simulink model "rlKinovaBallBalance"  (R2024a)
settings: Solver=ode15s  StartTime=0.0  StopTime=inf  MaxStep=0.005  RelTol=1e-4  AbsTol=1e-4
values from neighbouring files (symbols this model uses):
  max_torque = [3.5;    0.1;   0.75;    0.5]    [kinova_params.m]
  R1_q0 = 0    [kinova_params.m]
  R2_q0 = deg2rad(20)    [kinova_params.m]
  R3_q0 = 0    [kinova_params.m]
  R4_q0 = deg2rad(135)    [kinova_params.m]
  R5_q0 = 0    [kinova_params.m]
  R6_q0 = deg2rad(-65)    [kinova_params.m]
  R7_q0 = deg2rad(-90)    [kinova_params.m]
  U0 = [11.9 0.1 -1.4 0.09]    [kinova_params.m]
undefined symbols (not defined in the file or in its folder): Control, fluent0, L1, L2, L3, LS1, LS3, plate, R1, R2, R3, Rover, rover_path, RS1, RS3, Ts, vessel, X, Y, Z
libraries: sm_lib x253, nesl_utility x111, fl_lib x85, nesl_utility_internal x39, sdl_lib x20, ee_lib x10, simulink x6, mars_rover_lib x6, slpidlib x2, batteryecm_lib x2, robotalgslib x1, rllib x1
(part 11 of 12)

== system rlKinovaBallBalance/Kinova Ball Balance/Rover/Chassis/Roll and Steer/Steer/Steering Bracket L1 ==
  File Solid5 : sm_lib/Body Elements/File Solid  ExtGeomFileName=rover_chassis_steering_bracket.stl  UnitType=Custom  ExtGeomFileUnits=cm  StepReaderType=HEX  ExportConvexHullGeometry=off  InertiaType=CalculateFromGeometry  BasedOnType=Density  Density=1000  DensityUnits=kg/m^3  Mass=0  MassUnits=kg  CenterOfMass=[0 0 0]  CenterOfMassUnits=m  MomentsOfInertia=[1 1 1]*0  MomentsOfInertiaUnits=kg*m^2  ProductsOfInertia=[0 0 0]  ProductsOfInertiaUnits=kg*m^2  GraphicType=FromGeometry  MarkerShape=Sphere  MarkerSize=10  GraphicVisPropType=AdvancedVisualProperties  GraphicDiffuseColor=[0.2 0.2 0.2]  GraphicOpacity=1.0  GraphicSpecularColor=[1 1 1 1.0]  GraphicAmbientColor=[0.15 0.15 0.15 1.0]  GraphicEmissiveColor=[0.0 0.0 0.0 1.0]  GraphicShininess=90  DoExposeReferenceFrame=on  SerializedFrames=<Frames/>
  Reference Frame : sm_lib/Frames and Transforms/Reference Frame
  Rigid Transform : sm_lib/Frames and Transforms/Rigid Transform  RotationMethod=RotationMatrix  FollAlignAxisA=+X  BaseAlignAxisA=+Y  FollAlignAxisB=+Y  BaseAlignAxisB=+Z  RotationStandardAxis=+Z  RotationAngle=0.0  RotationAngleUnits=deg  RotationArbitraryAxis=[0 0 1]  RotationSequenceAxes=FollowerAxes  RotationSequence=XYX  RotationSequenceAngles=[0 0 0]  RotationSequenceAnglesUnits=deg  RotationMatrix=Rover.SteerBracket.SRJ_R  Quaternion=[1 0 0 0]  TranslationMethod=Cartesian  TranslationCartesianOffset=Rover.SteerBracket.SRJ_T  TranslationCartesianOffsetUnits=m  TranslationStandardAxis=+Z  TranslationStandardOffset=0  TranslationStandardOffsetUnits=m  TranslationROffset=0  TranslationROffsetUnits=m  TranslationThetaOffset=0  TranslationThetaOffsetUnits=deg  TranslationZOffset=0  TranslationZOffsetUnits=m
  Rigid Transform1 : sm_lib/Frames and Transforms/Rigid Transform  RotationMethod=RotationMatrix  FollAlignAxisA=+X  BaseAlignAxisA=+Y  FollAlignAxisB=+Y  BaseAlignAxisB=+Z  RotationStandardAxis=+Z  RotationAngle=0.0  RotationAngleUnits=deg  RotationArbitraryAxis=[0 0 1]  RotationSequenceAxes=FollowerAxes  RotationSequence=XYX  RotationSequenceAngles=[0 0 0]  RotationSequenceAnglesUnits=deg  RotationMatrix=Rover.SteerBracket.WRJ_R  Quaternion=[1 0 0 0]  TranslationMethod=Cartesian  TranslationCartesianOffset=Rover.SteerBracket.WRJ_T  TranslationCartesianOffsetUnits=m  TranslationStandardAxis=+Z  TranslationStandardOffset=0  TranslationStandardOffsetUnits=m  TranslationROffset=0  TranslationROffsetUnits=m  TranslationThetaOffset=0  TranslationThetaOffsetUnits=deg  TranslationZOffset=0  TranslationZOffsetUnits=m
  B : PMIOPort  Side=Left
  F : PMIOPort  Port=2  Side=Left
  connections:
  Rigid Transform/LConn1 -- Rigid Transform1/LConn1 -- Reference Frame/RConn1 -- File Solid5/RConn1
  F/RConn1 -- Rigid Transform1/RConn1
  Rigid Transform/RConn1 -- B/RConn1

== system rlKinovaBallBalance/Kinova Ball Balance/Rover/Chassis/Roll and Steer/Steer/Steering Bracket L3 ==
  File Solid5 : sm_lib/Body Elements/File Solid  ExtGeomFileName=rover_chassis_steering_bracket.stl  UnitType=Custom  ExtGeomFileUnits=cm  StepReaderType=HEX  ExportConvexHullGeometry=off  InertiaType=CalculateFromGeometry  BasedOnType=Density  Density=1000  DensityUnits=kg/m^3  Mass=0  MassUnits=kg  CenterOfMass=[0 0 0]  CenterOfMassUnits=m  MomentsOfInertia=[1 1 1]*0  MomentsOfInertiaUnits=kg*m^2  ProductsOfInertia=[0 0 0]  ProductsOfInertiaUnits=kg*m^2  GraphicType=FromGeometry  MarkerShape=Sphere  MarkerSize=10  GraphicVisPropType=AdvancedVisualProperties  GraphicDiffuseColor=[0.2 0.2 0.2]  GraphicOpacity=1.0  GraphicSpecularColor=[1 1 1 1.0]  GraphicAmbientColor=[0.15 0.15 0.15 1.0]  GraphicEmissiveColor=[0.0 0.0 0.0 1.0]  GraphicShininess=90  DoExposeReferenceFrame=on  SerializedFrames=<Frames/>
  Reference Frame : sm_lib/Frames and Transforms/Reference Frame
  Rigid Transform : sm_lib/Frames and Transforms/Rigid Transform  RotationMethod=RotationMatrix  FollAlignAxisA=+X  BaseAlignAxisA=+Y  FollAlignAxisB=+Y  BaseAlignAxisB=+Z  RotationStandardAxis=+Z  RotationAngle=0.0  RotationAngleUnits=deg  RotationArbitraryAxis=[0 0 1]  RotationSequenceAxes=FollowerAxes  RotationSequence=XYX  RotationSequenceAngles=[0 0 0]  RotationSequenceAnglesUnits=deg  RotationMatrix=Rover.SteerBracket.SRJ_R  Quaternion=[1 0 0 0]  TranslationMethod=Cartesian  TranslationCartesianOffset=Rover.SteerBracket.SRJ_T  TranslationCartesianOffsetUnits=m  TranslationStandardAxis=+Z  TranslationStandardOffset=0  TranslationStandardOffsetUnits=m  TranslationROffset=0  TranslationROffsetUnits=m  TranslationThetaOffset=0  TranslationThetaOffsetUnits=deg  TranslationZOffset=0  TranslationZOffsetUnits=m
  Rigid Transform1 : sm_lib/Frames and Transforms/Rigid Transform  RotationMethod=RotationMatrix  FollAlignAxisA=+X  BaseAlignAxisA=+Y  FollAlignAxisB=+Y  BaseAlignAxisB=+Z  RotationStandardAxis=+Z  RotationAngle=0.0  RotationAngleUnits=deg  RotationArbitraryAxis=[0 0 1]  RotationSequenceAxes=FollowerAxes  RotationSequence=XYX  RotationSequenceAngles=[0 0 0]  RotationSequenceAnglesUnits=deg  RotationMatrix=Rover.SteerBracket.WRJ_R  Quaternion=[1 0 0 0]  TranslationMethod=Cartesian  TranslationCartesianOffset=Rover.SteerBracket.WRJ_T  TranslationCartesianOffsetUnits=m  TranslationStandardAxis=+Z  TranslationStandardOffset=0  TranslationStandardOffsetUnits=m  TranslationROffset=0  TranslationROffsetUnits=m  TranslationThetaOffset=0  TranslationThetaOffsetUnits=deg  TranslationZOffset=0  TranslationZOffsetUnits=m
  B : PMIOPort  Side=Left
  F : PMIOPort  Port=2  Side=Right
  connections:
  File Solid5/RConn1 -- Reference Frame/RConn1 -- Rigid Transform/LConn1 -- Rigid Transform1/LConn1
  F/RConn1 -- Rigid Transform1/RConn1
  Rigid Transform/RConn1 -- B/RConn1

== system rlKinovaBallBalance/Kinova Ball Balance/Rover/Chassis/Roll and Steer/Steer/Steering Bracket R1 ==
  File Solid5 : sm_lib/Body Elements/File Solid  ExtGeomFileName=rover_chassis_steering_bracket.stl  UnitType=Custom  ExtGeomFileUnits=cm  StepReaderType=HEX  ExportConvexHullGeometry=off  InertiaType=CalculateFromGeometry  BasedOnType=Density  Density=1000  DensityUnits=kg/m^3  Mass=0  MassUnits=kg  CenterOfMass=[0 0 0]  CenterOfMassUnits=m  MomentsOfInertia=[1 1 1]*0  MomentsOfInertiaUnits=kg*m^2  ProductsOfInertia=[0 0 0]  ProductsOfInertiaUnits=kg*m^2  GraphicType=FromGeometry  MarkerShape=Sphere  MarkerSize=10  GraphicVisPropType=AdvancedVisualProperties  GraphicDiffuseColor=[0.2 0.2 0.2]  GraphicOpacity=1.0  GraphicSpecularColor=[1 1 1 1.0]  GraphicAmbientColor=[0.15 0.15 0.15 1.0]  GraphicEmissiveColor=[0.0 0.0 0.0 1.0]  GraphicShininess=90  DoExposeReferenceFrame=on  SerializedFrames=<Frames/>
  Reference Frame : sm_lib/Frames and Transforms/Reference Frame
  Rigid Transform : sm_lib/Frames and Transforms/Rigid Transform  RotationMethod=RotationMatrix  FollAlignAxisA=+X  BaseAlignAxisA=+Y  FollAlignAxisB=+Y  BaseAlignAxisB=+Z  RotationStandardAxis=+Z  RotationAngle=0.0  RotationAngleUnits=deg  RotationArbitraryAxis=[0 0 1]  RotationSequenceAxes=FollowerAxes  RotationSequence=XYX  RotationSequenceAngles=[0 0 0]  RotationSequenceAnglesUnits=deg  RotationMatrix=Rover.SteerBracket.SRJ_R  Quaternion=[1 0 0 0]  TranslationMethod=Cartesian  TranslationCartesianOffset=Rover.SteerBracket.SRJ_T  TranslationCartesianOffsetUnits=m  TranslationStandardAxis=+Z  TranslationStandardOffset=0  TranslationStandardOffsetUnits=m  TranslationROffset=0  TranslationROffsetUnits=m  TranslationThetaOffset=0  TranslationThetaOffsetUnits=deg  TranslationZOffset=0  TranslationZOffsetUnits=m
  Rigid Transform1 : sm_lib/Frames and Transforms/Rigid Transform  RotationMethod=RotationMatrix  FollAlignAxisA=+X  BaseAlignAxisA=+Y  FollAlignAxisB=+Y  BaseAlignAxisB=+Z  RotationStandardAxis=+Z  RotationAngle=0.0  RotationAngleUnits=deg  RotationArbitraryAxis=[0 0 1]  RotationSequenceAxes=FollowerAxes  RotationSequence=XYX  RotationSequenceAngles=[0 0 0]  RotationSequenceAnglesUnits=deg  RotationMatrix=Rover.SteerBracket.WRJ_R  Quaternion=[1 0 0 0]  TranslationMethod=Cartesian  TranslationCartesianOffset=Rover.SteerBracket.WRJ_T  TranslationCartesianOffsetUnits=m  TranslationStandardAxis=+Z  TranslationStandardOffset=0  TranslationStandardOffsetUnits=m  TranslationROffset=0  TranslationROffsetUnits=m  TranslationThetaOffset=0  TranslationThetaOffsetUnits=deg  TranslationZOffset=0  TranslationZOffsetUnits=m
  Transform Right Side : sm_lib/Frames and Transforms/Rigid Transform  RotationMethod=StandardAxis  FollAlignAxisA=+X  BaseAlignAxisA=+Y  FollAlignAxisB=+Y  BaseAlignAxisB=+Z  RotationStandardAxis=+Y  RotationAngle=180  RotationAngleUnits=deg  RotationArbitraryAxis=[0 0 1]  RotationSequenceAxes=FollowerAxes  RotationSequence=XYX  RotationSequenceAngles=[0 0 0]  RotationSequenceAnglesUnits=deg  RotationMatrix=[1 0 0; 0 1 0; 0 0 1]  Quaternion=[1 0 0 0]  TranslationMethod=None  TranslationCartesianOffset=[0 0 0]  TranslationCartesianOffsetUnits=m  TranslationStandardAxis=+Z  TranslationStandardOffset=0  TranslationStandardOffsetUnits=m  TranslationROffset=0  TranslationROffsetUnits=m  TranslationThetaOffset=0  TranslationThetaOffsetUnits=deg  TranslationZOffset=0  TranslationZOffsetUnits=m
  B : PMIOPort  Side=Right
  F : PMIOPort  Port=2  Side=Left
  connections:
  Rigid Transform/LConn1 -- Rigid Transform1/LConn1 -- Reference Frame/RConn1 -- File Solid5/RConn1
  Transform Right Side/RConn1 -- Rigid Transform1/RConn1
  Rigid Transform/RConn1 -- B/RConn1
  Transform Right Side/LConn1 -- F/RConn1

== system rlKinovaBallBalance/Kinova Ball Balance/Rover/Chassis/Roll and Steer/Steer/Steering Bracket R3 ==
  File Solid5 : sm_lib/Body Elements/File Solid  ExtGeomFileName=rover_chassis_steering_bracket.stl  UnitType=Custom  ExtGeomFileUnits=cm  StepReaderType=HEX  ExportConvexHullGeometry=off  InertiaType=CalculateFromGeometry  BasedOnType=Density  Density=1000  DensityUnits=kg/m^3  Mass=0  MassUnits=kg  CenterOfMass=[0 0 0]  CenterOfMassUnits=m  MomentsOfInertia=[1 1 1]*0  MomentsOfInertiaUnits=kg*m^2  ProductsOfInertia=[0 0 0]  ProductsOfInertiaUnits=kg*m^2  GraphicType=FromGeometry  MarkerShape=Sphere  MarkerSize=10  GraphicVisPropType=AdvancedVisualProperties  GraphicDiffuseColor=[0.2 0.2 0.2]  GraphicOpacity=1.0  GraphicSpecularColor=[1 1 1 1.0]  GraphicAmbientColor=[0.15 0.15 0.15 1.0]  GraphicEmissiveColor=[0.0 0.0 0.0 1.0]  GraphicShininess=90  DoExposeReferenceFrame=on  SerializedFrames=<Frames/>
  Reference Frame : sm_lib/Frames and Transforms/Reference Frame
  Rigid Transform : sm_lib/Frames and Transforms/Rigid Transform  RotationMethod=RotationMatrix  FollAlignAxisA=+X  BaseAlignAxisA=+Y  FollAlignAxisB=+Y  BaseAlignAxisB=+Z  RotationStandardAxis=+Z  RotationAngle=0.0  RotationAngleUnits=deg  RotationArbitraryAxis=[0 0 1]  RotationSequenceAxes=FollowerAxes  RotationSequence=XYX  RotationSequenceAngles=[0 0 0]  RotationSequenceAnglesUnits=deg  RotationMatrix=Rover.SteerBracket.SRJ_R  Quaternion=[1 0 0 0]  TranslationMethod=Cartesian  TranslationCartesianOffset=Rover.SteerBracket.SRJ_T  TranslationCartesianOffsetUnits=m  TranslationStandardAxis=+Z  TranslationStandardOffset=0  TranslationStandardOffsetUnits=m  TranslationROffset=0  TranslationROffsetUnits=m  TranslationThetaOffset=0  TranslationThetaOffsetUnits=deg  TranslationZOffset=0  TranslationZOffsetUnits=m
  Rigid Transform1 : sm_lib/Frames and Transforms/Rigid Transform  RotationMethod=RotationMatrix  FollAlignAxisA=+X  BaseAlignAxisA=+Y  FollAlignAxisB=+Y  BaseAlignAxisB=+Z  RotationStandardAxis=+Z  RotationAngle=0.0  RotationAngleUnits=deg  RotationArbitraryAxis=[0 0 1]  RotationSequenceAxes=FollowerAxes  RotationSequence=XYX  RotationSequenceAngles=[0 0 0]  RotationSequenceAnglesUnits=deg  RotationMatrix=Rover.SteerBracket.WRJ_R  Quaternion=[1 0 0 0]  TranslationMethod=Cartesian  TranslationCartesianOffset=Rover.SteerBracket.WRJ_T  TranslationCartesianOffsetUnits=m  TranslationStandardAxis=+Z  TranslationStandardOffset=0  TranslationStandardOffsetUnits=m  TranslationROffset=0  TranslationROffsetUnits=m  TranslationThetaOffset=0  TranslationThetaOffsetUnits=deg  TranslationZOffset=0  TranslationZOffsetUnits=m
  Transform Right Side : sm_lib/Frames and Transforms/Rigid Transform  RotationMethod=StandardAxis  FollAlignAxisA=+X  BaseAlignAxisA=+Y  FollAlignAxisB=+Y  BaseAlignAxisB=+Z  RotationStandardAxis=+Y  RotationAngle=180  RotationAngleUnits=deg  RotationArbitraryAxis=[0 0 1]  RotationSequenceAxes=FollowerAxes  RotationSequence=XYX  RotationSequenceAngles=[0 0 0]  RotationSequenceAnglesUnits=deg  RotationMatrix=[1 0 0; 0 1 0; 0 0 1]  Quaternion=[1 0 0 0]  TranslationMethod=None  TranslationCartesianOffset=[0 0 0]  TranslationCartesianOffsetUnits=m  TranslationStandardAxis=+Z  TranslationStandardOffset=0  TranslationStandardOffsetUnits=m  TranslationROffset=0  TranslationROffsetUnits=m  TranslationThetaOffset=0  TranslationThetaOffsetUnits=deg  TranslationZOffset=0  TranslationZOffsetUnits=m
  B : PMIOPort  Side=Right
  F : PMIOPort  Port=2  Side=Left
  connections:
  Rigid Transform/RConn1 -- B/RConn1
  Transform Right Side/RConn1 -- Rigid Transform1/RConn1
  File Solid5/RConn1 -- Reference Frame/RConn1 -- Rigid Transform1/LConn1 -- Rigid Transform/LConn1
  Transform Right Side/LConn1 -- F/RConn1

== system rlKinovaBallBalance/Kinova Ball Balance/Control/Chassis Control/Target Direction and Speed/hold/RoverStopTime/Enabled Subsystem1 ==
  In1 : Inport
  Enable : EnablePort
  Out1 : Outport
  wires:
  In1/1 -> Out1/1

== system rlKinovaBallBalance/Kinova Ball Balance/Rover/Chassis/Powertrain/Electrical/Drive/Sense tL1 ==
  Ideal Torque Sensor : fl_lib/Mechanical/Mechanical Sensors/Ideal Torque Sensor
  PS-Simulink Converter6 : nesl_utility/PS-Simulink Converter  PhysicalDomain=network_engine_domain  SubClassName=ps_output  LeftPortType=input  RightPortType=output  PseudoPeriodic=off  Frequencies=[]  VectorFormat=1-D array  Unit=inherit  AffineConversion=off
  C : PMIOPort  Side=Right
  R : PMIOPort  Port=2  Side=Left
  T : Outport
  wires:
  PS-Simulink Converter6/1 -> T/1
  connections:
  Ideal Torque Sensor/LConn1 -- R/RConn1
  Ideal Torque Sensor/RConn2 -- PS-Simulink Converter6/LConn1
  Ideal Torque Sensor/RConn1 -- C/RConn1

== system rlKinovaBallBalance/Kinova Ball Balance/Rover/Chassis/Powertrain/Electrical/Drive/Sense tL2 ==
  Ideal Torque Sensor : fl_lib/Mechanical/Mechanical Sensors/Ideal Torque Sensor
  PS-Simulink Converter6 : nesl_utility/PS-Simulink Converter  PhysicalDomain=network_engine_domain  SubClassName=ps_output  LeftPortType=input  RightPortType=output  PseudoPeriodic=off  Frequencies=[]  VectorFormat=1-D array  Unit=inherit  AffineConversion=off
  C : PMIOPort  Side=Right
  R : PMIOPort  Port=2  Side=Left
  T : Outport
  wires:
  PS-Simulink Converter6/1 -> T/1
  connections:
  Ideal Torque Sensor/RConn1 -- C/RConn1
  Ideal Torque Sensor/RConn2 -- PS-Simulink Converter6/LConn1
  Ideal Torque Sensor/LConn1 -- R/RConn1

== system rlKinovaBallBalance/Kinova Ball Balance/Rover/Chassis/Powertrain/Electrical/Drive/Sense tL3 ==
  Ideal Torque Sensor : fl_lib/Mechanical/Mechanical Sensors/Ideal Torque Sensor
  PS-Simulink Converter6 : nesl_utility/PS-Simulink Converter  PhysicalDomain=network_engine_domain  SubClassName=ps_output  LeftPortType=input  RightPortType=output  PseudoPeriodic=off  Frequencies=[]  VectorFormat=1-D array  Unit=inherit  AffineConversion=off
  R : PMIOPort  Side=Left
  C : PMIOPort  Port=2  Side=Right
  T : Outport
  wires:
  PS-Simulink Converter6/1 -> T/1
  connections:
  Ideal Torque Sensor/LConn1 -- R/RConn1
  Ideal Torque Sensor/RConn2 -- PS-Simulink Converter6/LConn1
  Ideal Torque Sensor/RConn1 -- C/RConn1

== system rlKinovaBallBalance/Kinova Ball Balance/Rover/Chassis/Powertrain/Electrical/Drive/Sense tR1 ==
  Ideal Torque Sensor : fl_lib/Mechanical/Mechanical Sensors/Ideal Torque Sensor
  PS-Simulink Converter6 : nesl_utility/PS-Simulink Converter  PhysicalDomain=network_engine_domain  SubClassName=ps_output  LeftPortType=input  RightPortType=output  PseudoPeriodic=off  Frequencies=[]  VectorFormat=1-D array  Unit=inherit  AffineConversion=off
  C : PMIOPort  Side=Right
  R : PMIOPort  Port=2  Side=Left
  T : Outport
  wires:
  PS-Simulink Converter6/1 -> T/1
  connections:
  Ideal Torque Sensor/RConn1 -- C/RConn1
  Ideal Torque Sensor/RConn2 -- PS-Simulink Converter6/LConn1
  Ideal Torque Sensor/LConn1 -- R/RConn1

== system rlKinovaBallBalance/Kinova Ball Balance/Rover/Chassis/Powertrain/Electrical/Drive/Sense tR2 ==
  Ideal Torque Sensor : fl_lib/Mechanical/Mechanical Sensors/Ideal Torque Sensor
  PS-Simulink Converter6 : nesl_utility/PS-Simulink Converter  PhysicalDomain=network_engine_domain  SubClassName=ps_output  LeftPortType=input  RightPortType=output  PseudoPeriodic=off  Frequencies=[]  VectorFormat=1-D array  Unit=inherit  AffineConversion=off
  C : PMIOPort  Side=Right
  R : PMIOPort  Port=2  Side=Left
  T : Outport
  wires:
  PS-Simulink Converter6/1 -> T/1
  connections:
  Ideal Torque Sensor/LConn1 -- R/RConn1
  Ideal Torque Sensor/RConn2 -- PS-Simulink Converter6/LConn1
  Ideal Torque Sensor/RConn1 -- C/RConn1

== system rlKinovaBallBalance/Kinova Ball Balance/Rover/Chassis/Powertrain/Electrical/Drive/Sense tR3 ==
  Ideal Torque Sensor : fl_lib/Mechanical/Mechanical Sensors/Ideal Torque Sensor
  PS-Simulink Converter6 : nesl_utility/PS-Simulink Converter  PhysicalDomain=network_engine_domain  SubClassName=ps_output  LeftPortType=input  RightPortType=output  PseudoPeriodic=off  Frequencies=[]  VectorFormat=1-D array  Unit=inherit  AffineConversion=off
  C : PMIOPort  Side=Right
  R : PMIOPort  Port=2  Side=Left
  T : Outport
  wires:
  PS-Simulink Converter6/1 -> T/1
  connections:
  Ideal Torque Sensor/RConn1 -- C/RConn1
  Ideal Torque Sensor/RConn2 -- PS-Simulink Converter6/LConn1
  Ideal Torque Sensor/LConn1 -- R/RConn1

== system rlKinovaBallBalance/Kinova Ball Balance/Rover/Chassis/Powertrain/Electrical/Drive/Sensor iL1 ==
  Current Sensor : fl_lib/Electrical/Electrical Sensors/Current Sensor
  PS-Simulink Converter3 : nesl_utility/PS-Simulink Converter  PhysicalDomain=network_engine_domain  SubClassName=ps_output  LeftPortType=input  RightPortType=output  PseudoPeriodic=off  Frequencies=[]  VectorFormat=1-D array  Unit=inherit  AffineConversion=off
  + : PMIOPort  Side=Left
  - : PMIOPort  Port=2  Side=Right
  i : Outport
  wires:
  PS-Simulink Converter3/1 -> i/1
  connections:
  PS-Simulink Converter3/LConn1 -- Current Sensor/RConn1
  Current Sensor/RConn2 -- -/RConn1
  +/RConn1 -- Current Sensor/LConn1

== system rlKinovaBallBalance/Kinova Ball Balance/Rover/Chassis/Powertrain/Electrical/Drive/Sensor iL2 ==
  Current Sensor : fl_lib/Electrical/Electrical Sensors/Current Sensor
  PS-Simulink Converter3 : nesl_utility/PS-Simulink Converter  PhysicalDomain=network_engine_domain  SubClassName=ps_output  LeftPortType=input  RightPortType=output  PseudoPeriodic=off  Frequencies=[]  VectorFormat=1-D array  Unit=inherit  AffineConversion=off
  + : PMIOPort  Side=Left
  - : PMIOPort  Port=2  Side=Right
  i : Outport
  wires:
  PS-Simulink Converter3/1 -> i/1
  connections:
  +/RConn1 -- Current Sensor/LConn1
  Current Sensor/RConn2 -- -/RConn1
  PS-Simulink Converter3/LConn1 -- Current Sensor/RConn1

== system rlKinovaBallBalance/Kinova Ball Balance/Rover/Chassis/Powertrain/Electrical/Drive/Sensor iL3 ==
  Current Sensor : fl_lib/Electrical/Electrical Sensors/Current Sensor
  PS-Simulink Converter3 : nesl_utility/PS-Simulink Converter  PhysicalDomain=network_engine_domain  SubClassName=ps_output  LeftPortType=input  RightPortType=output  PseudoPeriodic=off  Frequencies=[]  VectorFormat=1-D array  Unit=inherit  AffineConversion=off
  + : PMIOPort  Side=Left
  - : PMIOPort  Port=2  Side=Right
  i : Outport
  wires:
  PS-Simulink Converter3/1 -> i/1
  connections:
  +/RConn1 -- Current Sensor/LConn1
  Current Sensor/RConn2 -- -/RConn1
  PS-Simulink Converter3/LConn1 -- Current Sensor/RConn1

== system rlKinovaBallBalance/Kinova Ball Balance/Rover/Chassis/Powertrain/Electrical/Drive/Sensor iR1 ==
  Current Sensor : fl_lib/Electrical/Electrical Sensors/Current Sensor
  PS-Simulink Converter3 : nesl_utility/PS-Simulink Converter  PhysicalDomain=network_engine_domain  SubClassName=ps_output  LeftPortType=input  RightPortType=output  PseudoPeriodic=off  Frequencies=[]  VectorFormat=1-D array  Unit=inherit  AffineConversion=off
  + : PMIOPort  Side=Left
  - : PMIOPort  Port=2  Side=Right
  i : Outport
  wires:
  PS-Simulink Converter3/1 -> i/1
  connections:
  +/RConn1 -- Current Sensor/LConn1
  Current Sensor/RConn2 -- -/RConn1
  PS-Simulink Converter3/LConn1 -- Current Sensor/RConn1

== system rlKinovaBallBalance/Kinova Ball Balance/Rover/Chassis/Powertrain/Electrical/Drive/Sensor iR2 ==
  Current Sensor : fl_lib/Electrical/Electrical Sensors/Current Sensor
  PS-Simulink Converter3 : nesl_utility/PS-Simulink Converter  PhysicalDomain=network_engine_domain  SubClassName=ps_output  LeftPortType=input  RightPortType=output  PseudoPeriodic=off  Frequencies=[]  VectorFormat=1-D array  Unit=inherit  AffineConversion=off
  + : PMIOPort  Side=Left
  - : PMIOPort  Port=2  Side=Right
  i : Outport
  wires:
  PS-Simulink Converter3/1 -> i/1
  connections:
  PS-Simulink Converter3/LConn1 -- Current Sensor/RConn1
  Current Sensor/RConn2 -- -/RConn1
  +/RConn1 -- Current Sensor/LConn1

== system rlKinovaBallBalance/Kinova Ball Balance/Rover/Chassis/Powertrain/Electrical/Drive/Sensor iR3 ==
  Current Sensor : fl_lib/Electrical/Electrical Sensors/Current Sensor
  PS-Simulink Converter3 : nesl_utility/PS-Simulink Converter  PhysicalDomain=network_engine_domain  SubClassName=ps_output  LeftPortType=input  RightPortType=output  PseudoPeriodic=off  Frequencies=[]  VectorFormat=1-D array  Unit=inherit  AffineConversion=off
  + : PMIOPort  Side=Left
  - : PMIOPort  Port=2  Side=Right
  i : Outport
  wires:
  PS-Simulink Converter3/1 -> i/1
  connections:
  PS-Simulink Converter3/LConn1 -- Current Sensor/RConn1
  Current Sensor/RConn2 -- -/RConn1
  +/RConn1 -- Current Sensor/LConn1

== system rlKinovaBallBalance/Kinova Ball Balance/Rover/Chassis/Powertrain/Electrical/Power/Sensing Temperature ==
  PS-Simulink Converter : nesl_utility/PS-Simulink Converter  PhysicalDomain=network_engine_domain  SubClassName=ps_output  LeftPortType=input  RightPortType=output  PseudoPeriodic=off  Frequencies=[]  VectorFormat=1-D array  Unit=inherit  AffineConversion=off
  Temperature Sensor : fl_lib/Thermal/Thermal Sensors/Temperature Sensor  temperature_measure=foundation.enum.MeasurementReference.difference
  Thermal Reference : fl_lib/Thermal/Thermal Elements/Thermal Reference
  A : PMIOPort  Side=Left
  T : Outport
  wires:
  PS-Simulink Converter/1 -> T/1
  connections:
  Thermal Reference/LConn1 -- Temperature Sensor/RConn1
  Temperature Sensor/RConn2 -- PS-Simulink Converter/LConn1
  A/RConn1 -- Temperature Sensor/LConn1

== system rlKinovaBallBalance/Kinova Ball Balance/Rover/Chassis/Powertrain/Electrical/Steer/Sense T1 ==
  Ideal Torque Sensor : fl_lib/Mechanical/Mechanical Sensors/Ideal Torque Sensor
  PS-Simulink Converter6 : nesl_utility/PS-Simulink Converter  PhysicalDomain=network_engine_domain  SubClassName=ps_output  LeftPortType=input  RightPortType=output  PseudoPeriodic=off  Frequencies=[]  VectorFormat=1-D array  Unit=inherit  AffineConversion=off
  C : PMIOPort  Side=Right
  R : PMIOPort  Port=2  Side=Left
  T : Outport
  wires:
  PS-Simulink Converter6/1 -> T/1
  connections:
  Ideal Torque Sensor/LConn1 -- R/RConn1
  Ideal Torque Sensor/RConn2 -- PS-Simulink Converter6/LConn1
  Ideal Torque Sensor/RConn1 -- C/RConn1

== system rlKinovaBallBalance/Kinova Ball Balance/Rover/Chassis/Powertrain/Electrical/Steer/Sense tL3 ==
  Ideal Torque Sensor : fl_lib/Mechanical/Mechanical Sensors/Ideal Torque Sensor
  PS-Simulink Converter6 : nesl_utility/PS-Simulink Converter  PhysicalDomain=network_engine_domain  SubClassName=ps_output  LeftPortType=input  RightPortType=output  PseudoPeriodic=off  Frequencies=[]  VectorFormat=1-D array  Unit=inherit  AffineConversion=off
  C : PMIOPort  Side=Right
  R : PMIOPort  Port=2  Side=Left
  T : Outport
  wires:
  PS-Simulink Converter6/1 -> T/1
  connections:
  Ideal Torque Sensor/LConn1 -- R/RConn1
  Ideal Torque Sensor/RConn2 -- PS-Simulink Converter6/LConn1
  Ideal Torque Sensor/RConn1 -- C/RConn1

== system rlKinovaBallBalance/Kinova Ball Balance/Rover/Chassis/Powertrain/Electrical/Steer/Sense tR1 ==
  Ideal Torque Sensor : fl_lib/Mechanical/Mechanical Sensors/Ideal Torque Sensor
  PS-Simulink Converter6 : nesl_utility/PS-Simulink Converter  PhysicalDomain=network_engine_domain  SubClassName=ps_output  LeftPortType=input  RightPortType=output  PseudoPeriodic=off  Frequencies=[]  VectorFormat=1-D array  Unit=inherit  AffineConversion=off
  C : PMIOPort  Side=Right
  R : PMIOPort  Port=2  Side=Left
  T : Outport
  wires:
  PS-Simulink Converter6/1 -> T/1
  connections:
  Ideal Torque Sensor/RConn1 -- C/RConn1
  Ideal Torque Sensor/RConn2 -- PS-Simulink Converter6/LConn1
  Ideal Torque Sensor/LConn1 -- R/RConn1

== system rlKinovaBallBalance/Kinova Ball Balance/Rover/Chassis/Powertrain/Electrical/Steer/Sense tR3 ==
  Ideal Torque Sensor : fl_lib/Mechanical/Mechanical Sensors/Ideal Torque Sensor
  PS-Simulink Converter6 : nesl_utility/PS-Simulink Converter  PhysicalDomain=network_engine_domain  SubClassName=ps_output  LeftPortType=input  RightPortType=output  PseudoPeriodic=off  Frequencies=[]  VectorFormat=1-D array  Unit=inherit  AffineConversion=off
  C : PMIOPort  Side=Right
  R : PMIOPort  Port=2  Side=Left
  T : Outport
  wires:
  PS-Simulink Converter6/1 -> T/1
  connections:
  Ideal Torque Sensor/RConn1 -- C/RConn1
  Ideal Torque Sensor/RConn2 -- PS-Simulink Converter6/LConn1
  Ideal Torque Sensor/LConn1 -- R/RConn1

== system rlKinovaBallBalance/Kinova Ball Balance/Rover/Chassis/Powertrain/Electrical/Steer/Sensor iL1 ==
  Current Sensor : fl_lib/Electrical/Electrical Sensors/Current Sensor
  PS-Simulink Converter3 : nesl_utility/PS-Simulink Converter  PhysicalDomain=network_engine_domain  SubClassName=ps_output  LeftPortType=input  RightPortType=output  PseudoPeriodic=off  Frequencies=[]  VectorFormat=1-D array  Unit=inherit  AffineConversion=off
  + : PMIOPort  Side=Left
  - : PMIOPort  Port=2  Side=Right
  i : Outport
  wires:
  PS-Simulink Converter3/1 -> i/1
  connections:
  PS-Simulink Converter3/LConn1 -- Current Sensor/RConn1
  Current Sensor/RConn2 -- -/RConn1
  +/RConn1 -- Current Sensor/LConn1

== system rlKinovaBallBalance/Kinova Ball Balance/Rover/Chassis/Powertrain/Electrical/Steer/Sensor iL3 ==
  Current Sensor : fl_lib/Electrical/Electrical Sensors/Current Sensor
  PS-Simulink Converter3 : nesl_utility/PS-Simulink Converter  PhysicalDomain=network_engine_domain  SubClassName=ps_output  LeftPortType=input  RightPortType=output  PseudoPeriodic=off  Frequencies=[]  VectorFormat=1-D array  Unit=inherit  AffineConversion=off
  + : PMIOPort  Side=Left
  - : PMIOPort  Port=2  Side=Right
  i : Outport
  wires:
  PS-Simulink Converter3/1 -> i/1
  connections:
  +/RConn1 -- Current Sensor/LConn1
  Current Sensor/RConn2 -- -/RConn1
  PS-Simulink Converter3/LConn1 -- Current Sensor/RConn1

== system rlKinovaBallBalance/Kinova Ball Balance/Rover/Chassis/Powertrain/Electrical/Steer/Sensor iR1 ==
  Current Sensor : fl_lib/Electrical/Electrical Sensors/Current Sensor
  PS-Simulink Converter3 : nesl_utility/PS-Simulink Converter  PhysicalDomain=network_engine_domain  SubClassName=ps_output  LeftPortType=input  RightPortType=output  PseudoPeriodic=off  Frequencies=[]  VectorFormat=1-D array  Unit=inherit  AffineConversion=off
  + : PMIOPort  Side=Left
  - : PMIOPort  Port=2  Side=Right
  i : Outport
  wires:
  PS-Simulink Converter3/1 -> i/1
  connections:
  +/RConn1 -- Current Sensor/LConn1
  Current Sensor/RConn2 -- -/RConn1
  PS-Simulink Converter3/LConn1 -- Current Sensor/RConn1

== system rlKinovaBallBalance/Kinova Ball Balance/Rover/Chassis/Powertrain/Electrical/Steer/Sensor iR3 ==
  Current Sensor : fl_lib/Electrical/Electrical Sensors/Current Sensor
  PS-Simulink Converter3 : nesl_utility/PS-Simulink Converter  PhysicalDomain=network_engine_domain  SubClassName=ps_output  LeftPortType=input  RightPortType=output  PseudoPeriodic=off  Frequencies=[]  VectorFormat=1-D array  Unit=inherit  AffineConversion=off
  + : PMIOPort  Side=Left
  - : PMIOPort  Port=2  Side=Right
  i : Outport
  wires:
  PS-Simulink Converter3/1 -> i/1
  connections:
  PS-Simulink Converter3/LConn1 -- Current Sensor/RConn1
  Current Sensor/RConn2 -- -/RConn1
  +/RConn1 -- Current Sensor/LConn1

== system rlKinovaBallBalance/Kinova Ball Balance/Rover/Chassis/Powertrain/Ideal/Drive/Sense wL1 ==
  Ideal Rotational Motion Sensor : fl_lib/Mechanical/Mechanical Sensors/Ideal Rotational Motion Sensor  reference=foundation.enum.MeasurementReference.difference  acceleration_port=false  velocity_port=true  position_port=true  wrap_angle=simscape.enum.onoff.off  offset=0 rad
  PS Terminator : fl_lib/Physical Signals/Sinks/PS Terminator
  PS-Simulink Converter : nesl_utility/PS-Simulink Converter  PhysicalDomain=network_engine_domain  SubClassName=ps_output  LeftPortType=input  RightPortType=output  PseudoPeriodic=off  Frequencies=[]  VectorFormat=1-D array  Unit=inherit  AffineConversion=off
  R : PMIOPort  Side=Right
  C : PMIOPort  Port=2  Side=Left
  w : Outport
  wires:
  PS-Simulink Converter/1 -> w/1
  connections:
  Ideal Rotational Motion Sensor/RConn2 -- PS-Simulink Converter/LConn1
  Ideal Rotational Motion Sensor/LConn1 -- R/RConn1
  Ideal Rotational Motion Sensor/RConn1 -- C/RConn1
  Ideal Rotational Motion Sensor/RConn3 -- PS Terminator/LConn1

== system rlKinovaBallBalance/Kinova Ball Balance/Rover/Chassis/Powertrain/Ideal/Drive/Sense wL2 ==
  Ideal Rotational Motion Sensor : fl_lib/Mechanical/Mechanical Sensors/Ideal Rotational Motion Sensor  reference=foundation.enum.MeasurementReference.difference  acceleration_port=false  velocity_port=true  position_port=true  wrap_angle=simscape.enum.onoff.off  offset=0 rad
  PS Terminator : fl_lib/Physical Signals/Sinks/PS Terminator
  PS-Simulink Converter : nesl_utility/PS-Simulink Converter  PhysicalDomain=network_engine_domain  SubClassName=ps_output  LeftPortType=input  RightPortType=output  PseudoPeriodic=off  Frequencies=[]  VectorFormat=1-D array  Unit=inherit  AffineConversion=off
  R : PMIOPort  Side=Right
  C : PMIOPort  Port=2  Side=Left
  w : Outport
  wires:
  PS-Simulink Converter/1 -> w/1
  connections:
  Ideal Rotational Motion Sensor/RConn3 -- PS Terminator/LConn1
  Ideal Rotational Motion Sensor/RConn1 -- C/RConn1
  Ideal Rotational Motion Sensor/LConn1 -- R/RConn1
  Ideal Rotational Motion Sensor/RConn2 -- PS-Simulink Converter/LConn1

== system rlKinovaBallBalance/Kinova Ball Balance/Rover/Chassis/Powertrain/Ideal/Drive/Sense wL3 ==
  Ideal Rotational Motion Sensor : fl_lib/Mechanical/Mechanical Sensors/Ideal Rotational Motion Sensor  reference=foundation.enum.MeasurementReference.difference  acceleration_port=false  velocity_port=true  position_port=true  wrap_angle=simscape.enum.onoff.off  offset=0 rad
  PS Terminator : fl_lib/Physical Signals/Sinks/PS Terminator
  PS-Simulink Converter : nesl_utility/PS-Simulink Converter  PhysicalDomain=network_engine_domain  SubClassName=ps_output  LeftPortType=input  RightPortType=output  PseudoPeriodic=off  Frequencies=[]  VectorFormat=1-D array  Unit=inherit  AffineConversion=off
  R : PMIOPort  Side=Right
  C : PMIOPort  Port=2  Side=Left
  w : Outport
  wires:
  PS-Simulink Converter/1 -> w/1
  connections:
  Ideal Rotational Motion Sensor/RConn2 -- PS-Simulink Converter/LConn1
  Ideal Rotational Motion Sensor/LConn1 -- R/RConn1
  Ideal Rotational Motion Sensor/RConn1 -- C/RConn1
  Ideal Rotational Motion Sensor/RConn3 -- PS Terminator/LConn1

== system rlKinovaBallBalance/Kinova Ball Balance/Rover/Chassis/Powertrain/Ideal/Drive/Sense wR1 ==
  Ideal Rotational Motion Sensor : fl_lib/Mechanical/Mechanical Sensors/Ideal Rotational Motion Sensor  reference=foundation.enum.MeasurementReference.difference  acceleration_port=false  velocity_port=true  position_port=true  wrap_angle=simscape.enum.onoff.off  offset=0 rad
  PS Terminator : fl_lib/Physical Signals/Sinks/PS Terminator
  PS-Simulink Converter : nesl_utility/PS-Simulink Converter  PhysicalDomain=network_engine_domain  SubClassName=ps_output  LeftPortType=input  RightPortType=output  PseudoPeriodic=off  Frequencies=[]  VectorFormat=1-D array  Unit=inherit  AffineConversion=off
  R : PMIOPort  Side=Right
  C : PMIOPort  Port=2  Side=Left
  w : Outport
  wires:
  PS-Simulink Converter/1 -> w/1
  connections:
  Ideal Rotational Motion Sensor/RConn2 -- PS-Simulink Converter/LConn1
  Ideal Rotational Motion Sensor/LConn1 -- R/RConn1
  Ideal Rotational Motion Sensor/RConn1 -- C/RConn1
  Ideal Rotational Motion Sensor/RConn3 -- PS Terminator/LConn1

== system rlKinovaBallBalance/Kinova Ball Balance/Rover/Chassis/Powertrain/Ideal/Drive/Sense wR2 ==
  Ideal Rotational Motion Sensor : fl_lib/Mechanical/Mechanical Sensors/Ideal Rotational Motion Sensor  reference=foundation.enum.MeasurementReference.difference  acceleration_port=false  velocity_port=true  position_port=true  wrap_angle=simscape.enum.onoff.off  offset=0 rad
  PS Terminator : fl_lib/Physical Signals/Sinks/PS Terminator
  PS-Simulink Converter : nesl_utility/PS-Simulink Converter  PhysicalDomain=network_engine_domain  SubClassName=ps_output  LeftPortType=input  RightPortType=output  PseudoPeriodic=off  Frequencies=[]  VectorFormat=1-D array  Unit=inherit  AffineConversion=off
  R : PMIOPort  Side=Right
  C : PMIOPort  Port=2  Side=Left
  w : Outport
  wires:
  PS-Simulink Converter/1 -> w/1
  connections:
  Ideal Rotational Motion Sensor/RConn3 -- PS Terminator/LConn1
  Ideal Rotational Motion Sensor/RConn1 -- C/RConn1
  Ideal Rotational Motion Sensor/LConn1 -- R/RConn1
  Ideal Rotational Motion Sensor/RConn2 -- PS-Simulink Converter/LConn1

== system rlKinovaBallBalance/Kinova Ball Balance/Rover/Chassis/Powertrain/Ideal/Drive/Sense wR3 ==
  Ideal Rotational Motion Sensor : fl_lib/Mechanical/Mechanical Sensors/Ideal Rotational Motion Sensor  reference=foundation.enum.MeasurementReference.difference  acceleration_port=false  velocity_port=true  position_port=true  wrap_angle=simscape.enum.onoff.off  offset=0 rad
  PS Terminator : fl_lib/Physical Signals/Sinks/PS Terminator
  PS-Simulink Converter : nesl_utility/PS-Simulink Converter  PhysicalDomain=network_engine_domain  SubClassName=ps_output  LeftPortType=input  RightPortType=output  PseudoPeriodic=off  Frequencies=[]  VectorFormat=1-D array  Unit=inherit  AffineConversion=off
  R : PMIOPort  Side=Right
  C : PMIOPort  Port=2  Side=Left
  w : Outport
  wires:
  PS-Simulink Converter/1 -> w/1
  connections:
  Ideal Rotational Motion Sensor/RConn2 -- PS-Simulink Converter/LConn1
  Ideal Rotational Motion Sensor/LConn1 -- R/RConn1
  Ideal Rotational Motion Sensor/RConn1 -- C/RConn1
  Ideal Rotational Motion Sensor/RConn3 -- PS Terminator/LConn1

== system rlKinovaBallBalance/Kinova Ball Balance/Rover/Chassis/Powertrain/Ideal/Power/Sensing Temperature ==
  PS-Simulink Converter : nesl_utility/PS-Simulink Converter  PhysicalDomain=network_engine_domain  SubClassName=ps_output  LeftPortType=input  RightPortType=output  PseudoPeriodic=off  Frequencies=[]  VectorFormat=1-D array  Unit=inherit  AffineConversion=off
  Temperature Sensor : fl_lib/Thermal/Thermal Sensors/Temperature Sensor  temperature_measure=foundation.enum.MeasurementReference.difference
  Thermal Reference : fl_lib/Thermal/Thermal Elements/Thermal Reference
  A : PMIOPort  Side=Left
  T : Outport
  wires:
  PS-Simulink Converter/1 -> T/1
  connections:
  Thermal Reference/LConn1 -- Temperature Sensor/RConn1
  Temperature Sensor/RConn2 -- PS-Simulink Converter/LConn1
  A/RConn1 -- Temperature Sensor/LConn1

== system rlKinovaBallBalance/Kinova Ball Balance/Rover/Chassis/Powertrain/Ideal/Steer/Sense wL1 ==
  Ideal Rotational Motion Sensor : fl_lib/Mechanical/Mechanical Sensors/Ideal Rotational Motion Sensor  reference=foundation.enum.MeasurementReference.difference  acceleration_port=false  velocity_port=true  position_port=true  wrap_angle=simscape.enum.onoff.off  offset=0 rad
  PS Terminator : fl_lib/Physical Signals/Sinks/PS Terminator
  PS-Simulink Converter : nesl_utility/PS-Simulink Converter  PhysicalDomain=network_engine_domain  SubClassName=ps_output  LeftPortType=input  RightPortType=output  PseudoPeriodic=off  Frequencies=[]  VectorFormat=1-D array  Unit=inherit  AffineConversion=off
  R : PMIOPort  Side=Right
  C : PMIOPort  Port=2  Side=Left
  w : Outport
  wires:
  PS-Simulink Converter/1 -> w/1
  connections:
  Ideal Rotational Motion Sensor/RConn2 -- PS-Simulink Converter/LConn1
  Ideal Rotational Motion Sensor/LConn1 -- R/RConn1
  Ideal Rotational Motion Sensor/RConn1 -- C/RConn1
  Ideal Rotational Motion Sensor/RConn3 -- PS Terminator/LConn1

== system rlKinovaBallBalance/Kinova Ball Balance/Rover/Chassis/Powertrain/Ideal/Steer/Sense wL3 ==
  Ideal Rotational Motion Sensor : fl_lib/Mechanical/Mechanical Sensors/Ideal Rotational Motion Sensor  reference=foundation.enum.MeasurementReference.difference  acceleration_port=false  velocity_port=true  position_port=true  wrap_angle=simscape.enum.onoff.off  offset=0 rad
  PS Terminator : fl_lib/Physical Signals/Sinks/PS Terminator
  PS-Simulink Converter : nesl_utility/PS-Simulink Converter  PhysicalDomain=network_engine_domain  SubClassName=ps_output  LeftPortType=input  RightPortType=output  PseudoPeriodic=off  Frequencies=[]  VectorFormat=1-D array  Unit=inherit  AffineConversion=off
  R : PMIOPort  Side=Right
  C : PMIOPort  Port=2  Side=Left
  w : Outport
  wires:
  PS-Simulink Converter/1 -> w/1
  connections:
  Ideal Rotational Motion Sensor/RConn2 -- PS-Simulink Converter/LConn1
  Ideal Rotational Motion Sensor/LConn1 -- R/RConn1
  Ideal Rotational Motion Sensor/RConn1 -- C/RConn1
  Ideal Rotational Motion Sensor/RConn3 -- PS Terminator/LConn1

== system rlKinovaBallBalance/Kinova Ball Balance/Rover/Chassis/Powertrain/Ideal/Steer/Sense wR1 ==
  Ideal Rotational Motion Sensor : fl_lib/Mechanical/Mechanical Sensors/Ideal Rotational Motion Sensor  reference=foundation.enum.MeasurementReference.difference  acceleration_port=false  velocity_port=true  position_port=true  wrap_angle=simscape.enum.onoff.off  offset=0 rad
  PS Terminator : fl_lib/Physical Signals/Sinks/PS Terminator
  PS-Simulink Converter : nesl_utility/PS-Simulink Converter  PhysicalDomain=network_engine_domain  SubClassName=ps_output  LeftPortType=input  RightPortType=output  PseudoPeriodic=off  Frequencies=[]  VectorFormat=1-D array  Unit=inherit  AffineConversion=off
  R : PMIOPort  Side=Right
  C : PMIOPort  Port=2  Side=Left
  w : Outport
  wires:
  PS-Simulink Converter/1 -> w/1
  connections:
  Ideal Rotational Motion Sensor/RConn2 -- PS-Simulink Converter/LConn1
  Ideal Rotational Motion Sensor/LConn1 -- R/RConn1
  Ideal Rotational Motion Sensor/RConn1 -- C/RConn1
  Ideal Rotational Motion Sensor/RConn3 -- PS Terminator/LConn1

== system rlKinovaBallBalance/Kinova Ball Balance/Rover/Chassis/Powertrain/Ideal/Steer/Sense wR3 ==
  Ideal Rotational Motion Sensor : fl_lib/Mechanical/Mechanical Sensors/Ideal Rotational Motion Sensor  reference=foundation.enum.MeasurementReference.difference  acceleration_port=false  velocity_port=true  position_port=true  wrap_angle=simscape.enum.onoff.off  offset=0 rad
  PS Terminator : fl_lib/Physical Signals/Sinks/PS Terminator
  PS-Simulink Converter : nesl_utility/PS-Simulink Converter  PhysicalDomain=network_engine_domain  SubClassName=ps_output  LeftPortType=input  RightPortType=output  PseudoPeriodic=off  Frequencies=[]  VectorFormat=1-D array  Unit=inherit  AffineConversion=off
  R : PMIOPort  Side=Right
  C : PMIOPort  Port=2  Side=Left
  w : Outport
  wires:
  PS-Simulink Converter/1 -> w/1
  connections:
  Ideal Rotational Motion Sensor/RConn2 -- PS-Simulink Converter/LConn1
  Ideal Rotational Motion Sensor/LConn1 -- R/RConn1
  Ideal Rotational Motion Sensor/RConn1 -- C/RConn1
  Ideal Rotational Motion Sensor/RConn3 -- PS Terminator/LConn1

== matlab function rlKinovaBallBalance/Kinova Ball Balance/Observation/MATLAB Function ==
  data: qPlate input; R_W2vessel output
function R_W2vessel = quatToR_W2vessel(qPlate)
    q = qPlate(:).';
    n = norm(q);
    if n == 0, R_W2vessel = eye(3); 
        return; 
    end
    q = q / n;

    % Матрица body->world
    w=q(1); x=q(2); y=q(3); z=q(4);
    R_bw = [1-2*(y*y+z*z), 2*(x*y - w*z), 2*(x*z + w*y);
            2*(x*y + w*z), 1-2*(x*x+z*z), 2*(y*z - w*x);
            2*(x*z - w*y), 2*(y*z + w*x), 1-2*(x*x+y*y)];
    % world->vessel
    R_W2vessel = R_bw.';
end

== matlab function rlKinovaBallBalance/MATLAB Function ==
  data: u input double size=[14 1]; y output double size=[13 1]
% function y = fcn(u)
%     % ---------- константы ----------
%     NSTATE   = coder.const(12);
%     NPOSE    = coder.const(13);
%     MAXRETRY = coder.const(500);
%     DTWAIT   = 2;                       % c
%     % ---------- вывод по умолчанию ----------
%     persistent prevState
%     if isempty(prevState); prevState = zeros(1,NSTATE,'double'); end
%     y      = prevState;                 % держим старое, пока нет данных
%     % ---------- пути (persistent) -----------
%     persistent wd feedDat feedOk poseDat poseOk resetOk fidLog stepCnt
%     if isempty(wd)
%     wd      = '/home/dika/Documents/sloshing_balance_via_roboarm/rlKinova_marsRover_fluent_via_files/data/work_dir/';
%     feedDat = [wd 'feed.dat'];
%     feedOk  = [wd 'feed.ok'];
%     poseDat = [wd 'pose.dat'];
%     poseOk  = [wd 'pose.ok'];
%     resetOk = '/home/dika/Documents/sloshing_balance_via_roboarm/glass_liquid_sloshing_simulink/vessel-res-2/reset/reset.ok';
%     fidLog  = -1;  % безопасное значение
%     stepCnt = int32(0);
%     end
%     % ---------- ждём feed.ok (НЕ трогаем u) ----------
%     coder.extrinsic('exist','pause','delete');   % для Normal/Accel
%     retry = 0;
%     while ~exist(feedOk,'file') && retry < MAXRETRY
%     pause(DTWAIT);
%     retry = retry + 1;
%     end
%     if retry == MAXRETRY
%     return;     % тайм-аут → enable=false, возвращаем предыдущее y
%     end
%     % ---------- читаем feed.dat ----------
%     fid = fopen(feedDat,'r');
%     state = zeros(1,NSTATE,'double');
%     for k = 1:NSTATE
%     state(k) = fscanf(fid,'%f',1);
%     end
%     fclose(fid);
%     y = state;          % отдаём наблюдение наверх
%     prevState = state;  % запоминаем для следующего цикла
%     % ---------- файл-флаг снимаем ----------
%     delete(feedOk);     % signal to Fluent that we consumed data
%     % ---------- пишем pose.dat (используем вход u ТОЛЬКО ЗДЕСЬ) ----------
%     pose = u(1:NPOSE);
%     fid  = fopen(poseDat,'w');
%     for k = 1:NPOSE
%     fprintf(fid,'%.6f ', pose(k));   % ← scalar
%     end
%     fprintf(fid,'\n');
%     fclose(fid);
%     fclose(fopen(poseOk,'w'));   % создаём pose.ok
%     % ---------- лог ----------
%     stepCnt = stepCnt + 1;
%     if fidLog < 0 || ~isnumeric(fidLog)
%     fidLog = fopen([wd 'rl_log.txt'],'a');
%     end
%     if fidLog >= 0  && mod(stepCnt, 5) == 0
%     fprintf(fidLog,'step %6d  vx=%.3f vy=%.3f  vz=%.3f wx=%.3f wy=%.3f wz=%.3f\n',...
%     stepCnt, pose(8), pose(9), pose(10), pose(11), pose(12), pose(13));
%     fclose(fidLog);
%     fidLog = -1;
%     end
%     % ---------- обработка reset-флага (после enable) ----------
%     if u(NPOSE+1) > 0
%     fclose(fopen(resetOk,'w'));
%     end
% end

function y = fcn(u)
% ---------- константы ----------
NSTATE   = coder.const(13);   % должно совпадать с количеством чисел в feed.dat
NPOSE    = coder.const(13);   % [r(3); q(4); v(3); w(3)] = 13
MAXRETRY = coder.const(500);
DTWAIT   = 2;                 % c

% ---------- вывод по умолчанию ----------
persistent prevState
if isempty(prevState)
    prevState = zeros(NSTATE,1,'double');  % колонка
end
y = prevState;

% ---------- пути (persistent) -----------
persistent wd feedDat feedOk poseDat poseOk resetOk stepCnt handshaked
if isempty(wd)
    wd         = '/home/dika/Documents/sloshing_balance_via_roboarm/rlKinova_marsRover_fluent_via_files/data/work_dir/';
    feedDat    = [wd 'feed.dat'];
    feedOk     = [wd 'feed.ok'];
    poseDat    = [wd 'pose.dat'];
    poseOk     = [wd 'pose.ok'];
    resetOk    = '/home/dika/Documents/sloshing_balance_via_roboarm/glass_liquid_sloshing_simulink/vessel-res-2/reset/reset.ok';
    stepCnt    = int32(0);
    handshaked = false;
end

% --- extrinsic (I/O и паузы) ---
coder.extrinsic('exist','pause','delete','fopen','fclose','fprintf','fscanf');

% ---------- если ПЕРВЫЙ ТИК: публикуем позу и выходим ----------
if ~handshaked
    pose = reshape(u(1:NPOSE), [NPOSE 1]);
    fid = fopen(poseDat,'w');    
    fprintf(fid,'%.6f ', pose);
    fprintf(fid,'\n');
    fclose(fid);
    fid2 = fopen(poseOk,'w');   
    fclose(fid2);
    disp(handshaked);
    handshaked = true;
    return;  % y = prevState
end

% ---------- ждём feed.ok ----------
retry = 0;
while ~exist(feedOk,'file') && retry < MAXRETRY
    pause(DTWAIT);
    retry = retry + 1;
end
if retry == MAXRETRY
    return;  % отдаём предыдущее
end

% ---------- читаем feed.dat -> state [13x1] ----------
state = zeros(NSTATE,1,'double');
fid = fopen(feedDat,'r');   
for k = 1:NSTATE
    val = fscanf(fid,'%f',1);
    if isempty(val)
        break;
    end
    state(k) = val;
end
fclose(fid);

% ---------- отдаём наблюдение наверх ----------
y = reshape(state,[NSTATE 1]);
prevState = y;

% ---------- снять feed.ok ----------
if exist(feedOk,'file')
    delete(feedOk);
end

% ---------- публикуем текущую позу ----------
pose = reshape(u(1:NPOSE), [NPOSE 1]);
fid = fopen(poseDat,'w');         
fprintf(fid,'%.6f ', pose);
fprintf(fid,'\n');
fclose(fid);
fid2 = fopen(poseOk,'w');        
fclose(fid2);

% ---------- лог каждые 5 шагов ----------
stepCnt = stepCnt + 1;
if mod(stepCnt,5) == 0
    fidL = fopen([wd 'rl_log.txt'],'a'); 
    fprintf(fidL,'step %6d  vx=%.3f vy=%.3f vz=%.3f  wx=%.3f wy=%.3f wz=%.3f\n',...
        stepCnt, pose(8), pose(9), pose(10), pose(11), pose(12), pose(13));
    fclose(fidL);
end

% ---------- обработка reset-флага ----------
% reset-флаг идёт 14-м элементом входа
if numel(u) >= NPOSE+1 && u(NPOSE+1) > 0
    fidr = fopen(resetOk,'w');  
    fclose(fidr);
    handshaked = false;
end
end

== matlab function rlKinovaBallBalance/Kinova Ball Balance/Control/Chassis Control/Ackerman Steer Angle/Ackerman Steering Angle Formulation ==
  data: delta input; qSteerL3 output; L input; qSteerR3 output; d input; R output; L_R output; R_R output
function [qSteerL3,qSteerR3,R,L_R,R_R] = fcn(delta,L,d)
% Function to compute ackerman steering angles 
% from a bicycle steer angle.

R = L/tand(abs(delta));

if delta < 0
    qSteerL3 = atan2d(L,(R+d/2));
    qSteerR3 = atan2d(L,(R-d/2));
    L_R = (R+d/2);
    R_R = (R-d/2);
else
    qSteerL3 = -atan2d(L,(R-d/2));
    qSteerR3 = -atan2d(L,(R+d/2));
    L_R = (R-d/2);
    R_R = (R+d/2);
end

end

== matlab function rlKinovaBallBalance/Kinova Ball Balance/Control/Chassis Control/Chassis Velocity To Wheel Speed ==
  data: vTarget input; steer_ang input; A3_ROC input; L3_ROC input; R3_ROC input; wL1 output; wheel_r input; wL2 output; wL3 output; L input; wR1 output; wR2 output; wR3 output
function [wL1,wL2,wL3, wR1,wR2,wR3] = ...
    fcn(vTarget,steer_ang,A3_ROC,L3_ROC,R3_ROC,wheel_r,L)
% Function to compute wheel speed from a desired linear velocity and
% desired path.

if any(abs(steer_ang) > 0)

    wL1 = (vTarget/wheel_r)*sqrt(L3_ROC^2 + L^2)/A3_ROC;
    wL2 = vTarget * L3_ROC/(A3_ROC*wheel_r);
    wL3 = (vTarget/wheel_r)*sqrt(L3_ROC^2 + L^2)/A3_ROC;
    wR1 = (vTarget/wheel_r)*sqrt(R3_ROC^2 + L^2)/A3_ROC;
    wR2 = vTarget * R3_ROC/(A3_ROC*wheel_r);
    wR3 = (vTarget/wheel_r)*sqrt(R3_ROC^2 + L^2)/A3_ROC;

else
    wL1 = vTarget / wheel_r;
    wL2 = vTarget / wheel_r;
    wL3 = vTarget / wheel_r;
    wR1 = vTarget / wheel_r;
    wR2 = vTarget / wheel_r;
    wR3 = vTarget / wheel_r;
end

end

== matlab function rlKinovaBallBalance/Kinova Ball Balance/Control/Chassis Control/Target Dir To Bicycle Steer Angle/Rad2Deg ==
  data: u input; y output
function y = fcn(u)
y = rad2deg(u);

== matlab function rlKinovaBallBalance/Kinova Ball Balance/Control/Chassis Control/Target Direction and Speed/Trapezoidal Vel Profile ==
  data: t input; startTime input; accel input; deaccelStartTime input; linVel input; lin_Vel_out output
function lin_Vel_out = fcn(t,startTime,accel,deaccelStartTime,linVel)
% Function to create a trapezoidal profile for rover's desired linear
% velocity

t2 = linVel/accel + startTime;
t3 = deaccelStartTime + 0.2;
tf = linVel/accel + t3;

if t>=startTime && t<t2 
    lin_Vel_out = accel*(t-startTime);

elseif t>=t2 && t < t3 
    lin_Vel_out = linVel;

elseif t>= t3 && t < tf 
    lin_Vel_out = linVel-accel*(t-t3);

else
    lin_Vel_out = 0;    
end


end
